simulink model "espacioEstados"  (R2020b)
settings: Solver=VariableStepAuto  StartTime=0.0  StopTime=2  RelTol=1e-3
values from neighbouring files (symbols this model uses):
  B = 14.41e-6    (= 1.441e-05)    [parametros.m]
  J = 80.7e-6    (= 8.07e-05)    [parametros.m]
  K = 0.0879    [parametros.m]
  La = 1.5e-3    (= 0.0015)    [parametros.m]
  Ra = 8.3    [parametros.m]
settings Model: Creator=petir  LastModifiedBy=petir

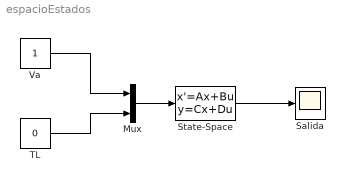
== system espacioEstados ==
  Mux : Mux  Inputs=2
  Salida : Scope
  State-Space : StateSpace  A=[-Ra/La -K/La; K/J -B/J]  B=[1/La 0; 0 -1/J]  C=[0 1]  D=[0 0]  InitialCondition=0
  TL : Constant  Value=0
  Va : Constant
  wires:
  Mux/1 -> State-Space/1
  Va/1 -> Mux/1
  TL/1 -> Mux/2
  State-Space/1 -> Salida/1
